simulink model "MPC_DUE"  (R2019a)
settings: Solver=FixedStepAuto  StartTime=0.0  StopTime=120  RelTol=1e-3  EnableMultiTasking=on
undefined symbols (not defined in the file or in its folder): DiscIntNeverNeededParam, i0, sigbuilder_block, Ts, u0, y0
libraries: MagnetoLibrary x3
settings Model: SimulationMode=external  ExtModeTrigDuration=2  Creator=jakub  LastModifiedBy=jakub
settings OptimizationCC: EnhancedBackFolding=on  PassReuseOutputArgsAs=Individual arguments  MaxStackSize=64  OptimizeBlockOrder=speed  DifferentSizesBufferReuse=on  OptimizationCustomize=off
settings DebuggingCC: ParameterTunabilityLossMsg=error
settings HardwareCC: ProdBitPerPointer=32  ProdBitPerSizeT=32  ProdBitPerPtrDiffT=32  ProdLargestAtomicInteger=Long  ProdLargestAtomicFloat=Double  ProdWordSize=32  ProdHWDeviceType=ARM Compatible->ARM Cortex
settings SFSimCC: MATLABDynamicMemAlloc=off
settings RTWCC: SystemTargetFile=ert.tlc  HardwareBoard=Arduino Due  TLCOptions=-aInlineSetEventsForThisBaseRateFcn=TLC_FALSE -aSuppressMultiTaskScheduler=TLC_FALSE -aRateBasedStepFcn=1  TemplateMakefile=ert_default_tmf  GenerateReport=on  Toolchain=Arduino ARM  BuildConfiguration=Faster Runs  IncludeHyperlinkInReport=on  LaunchReport=on  GenerateTraceInfo=on  GenerateTraceReport=on  GenerateTraceReportSl=on  GenerateTraceReportSf=on  GenerateTraceReportEml=on
settings CodeAppCC: ForceParamTrailComments=on  IgnoreCustomStorageClasses=off  OperatorAnnotations=on  SimulinkDataObjDesc=on  SFDataObjDesc=on  InsertBlockDesc=on
settings ERTTargetCC: SupportContinuousTime=on  SupportVariableSizeSignals=on  ExtModeStaticAllocSize=24576

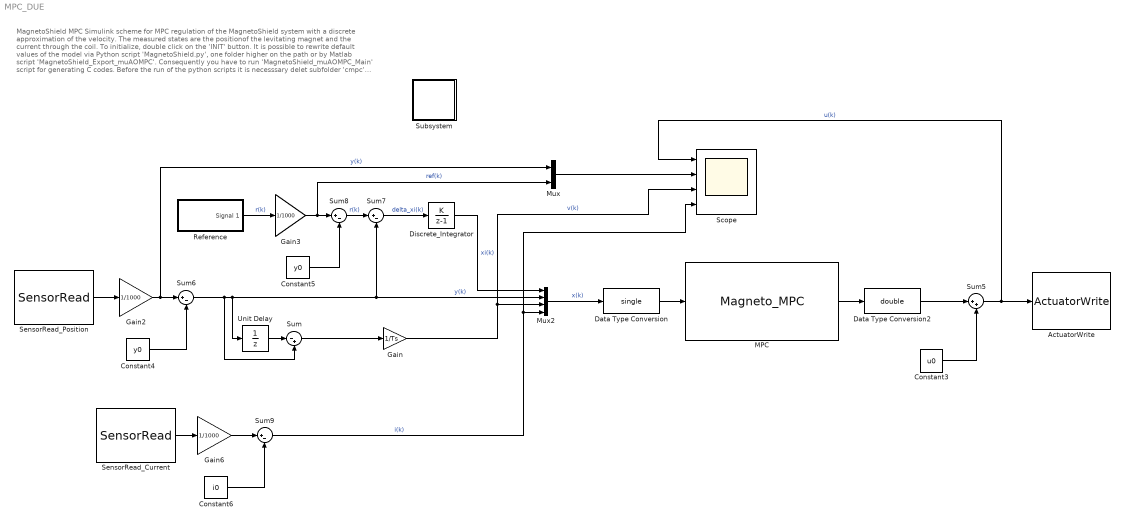
== system MPC_DUE ==
  note: MagnetoShield MPC
      | Simulink scheme for MPC regulation of the MagnetoShield system with a discrete approximation of the velocity.
      | The measured states are the positionof the levitating magnet and the current through the coil.
      | To initialize, double click on the 'INIT' button.
      |
      | It is possible to rewrite default values of the model via Python script 'MagnetoShield.py', one folder higher on
      | the path or by Matlab script 'MagnetoShield_Export_muAOMPC'.
      | Consequently you have to run 'MagnetoShield_muAOMPC_Main' script for generating C codes. Before the run
      | of the python scripts it is necesssary delet subfolder 'cmpc' (will be regenerated). If the application performance
      | did not change, errase all files in the subfolder '.../MagnetoShield_MPC_DUE/MagnetoShield_MPC_Control' too
      | and in 'MPC' block build the S-Function again.
      |
      | For a correct performance of the control-loop it is necessary to have '.../MagnetoShield_MPC_DUE/cmpc' folder
      | added in the Matlab path.
  ActuatorWrite : MagnetoLibrary/ActuatorWrite  Board=DUE  Units=Volts
      settings: SourceProductName=AutomationShield
  Constant3 : Constant  Value=u0
  Constant4 : Constant  Value=y0
  Constant5 : Constant  Value=y0
  Constant6 : Constant  Value=i0
  Data Type Conversion : DataTypeConversion  OutDataTypeStr=single
  Data Type Conversion2 : DataTypeConversion  OutDataTypeStr=double
  Discrete_Integrator : DiscreteIntegrator  IntegratorMethod=Accumulation: Forward Euler  SampleTime=Ts  LimitOutput=on  UpperSaturationLimit=100  LowerSaturationLimit=-100  ICPrevOutput=DiscIntNeverNeededParam  ICPrevScaledInput=DiscIntNeverNeededParam
  Gain : Gain  Gain=1/Ts
  Gain2 : Gain  Gain=1/1000
  Gain3 : Gain  Gain=1/1000
  Gain6 : Gain  Gain=1/1000
  MPC : S-Function  InitFcn=try, set_param(gcb,'FunctionName','Magneto_MPC'), end  FunctionName=Magneto_MPC  SFunctionModules=Magneto_MPC_wrapper mtx_ops mpc_const mpc mpc_ref mpc_stc mpc_inc fip_ops  SFunctionDeploymentMode=off  EnableBusSupport=off  mask(S-Function Builder){}
      mask help: Simulink:masks:SFunctionBuilder_MD
      mask init:
      | val = [[.9  0.75 0.75 1 1 .9 .9 1]',[1 1 0.75 0.75 .9 .9 1 .9]'];try , sys = get_param(gcb,'SfunBuilderFcnName');if isempty(sys), sys = get_param(gcb,'FunctionName'); end,catch, sys = get_param(gcb,'FunctionName'); end
      settings: CopyFcn=set_param(gcbh,'LinkStatus','none')  PreSaveFcn=try, set_param(gcb,'FunctionName','Magneto_MPC'), end  OpenFcn=sfunctionwizard(gcbh)
      mask Display: plot(val(:,1),val(:,2)),disp(sys), port_label('input',1,'u'), port_label('output',1,'y')
  Mux : Mux  Inputs=2
  Mux2 : Mux
  Reference : Subsystem  Tag=STV Subsys  LoadFcn=sigbuilder_block('load');  StartFcn=sigbuilder_block('start');  StopFcn=sigbuilder_block('stop');  ClipboardFcn=sigbuilder_block('clipboard');  mask(Sigbuilder block){tuvar=[0:10]}
      mask help: Simulink:masks:SigbuilderBlock_MD
      mask init:
      | if ~strcmp(get_param(bdroot(gcbh),'SimulationStatus'),'stopped') tuvar = sigbuilder_block('maskInit'); end
      settings: CopyFcn=sigbuilder_block('copy');  DeleteFcn=sigbuilder_block('delete');  ModelCloseFcn=sigbuilder_block('modelClose');  PreSaveFcn=sigbuilder_block('preSave');  PauseFcn=sigbuilder_block('pause');  ContinueFcn=sigbuilder_block('continue');  NameChangeFcn=sigbuilder_block('namechange');  OpenFcn=sigbuilder_block('open',[61.8 52.2 1012.8 447.6 ]);  CloseFcn=sigbuilder_block('close');
      mask Display: plot(0, 0, 100, 100,[2, 2, 32, 32, 2], [68, 8, 8, 68, 68],[32, 2], [38, 38], [32, 19, 2],[53, 60, 44], [32, 17, 17, 2],[16, 16, 31, 31]);txt = getActiveGroup(gcbh);text(2, 100, txt,'verticalAlignment', 'top');
  Scope : Scope  NumInputPorts=4
  SensorRead_Current : MagnetoLibrary/SensorRead  board=DUE  sensor=Current [mA]  sampling=Ts
      settings: SourceProductName=AutomationShield
  SensorRead_Position : MagnetoLibrary/SensorRead  board=DUE  sensor=Distance [mm]  sampling=Ts
      settings: SourceProductName=AutomationShield
  Subsystem : Subsystem
      settings: OpenFcn=|
      | clear;close all;clc;
      | cd(fileparts(which(gcs)));
      | load '../../../../../../matlab/examples/MagnetoShield/MagnetoShield_Models_Greybox_SS';
      | 
      | Ts = 0.003
      mask Display: disp('INIT')
  Sum : Sum  Inputs=|-+
  Sum5 : Sum  Inputs=|++
  Sum{6..9} (4 alike) : Sum  Inputs=|+-
  Unit Delay : UnitDelay  SampleTime=-1  HasFrameUpgradeWarning=on
  wires:
  SensorRead_Current/1 -> Gain6/1
  Discrete_Integrator/1 -> Mux2/1  "xi(k)"
  Unit Delay/1 -> Sum/1
  Sum/1 -> Gain/1
  Gain3/1 -> Mux/2, Sum8/1  "ref(k)"
  Constant5/1 -> Sum8/2
  Constant6/1 -> Sum9/2
  Gain/1 -> Mux2/3, Scope/3  "v(k)"
  Reference/1(Signal 1) -> Gain3/1  "r(k)"
  Sum8/1 -> Sum7/1  "r(k)"
  Constant4/1 -> Sum6/2
  Sum7/1 -> Discrete_Integrator/1  "delta_xi(k)"
  Gain2/1 -> Mux/1, Sum6/1  "y(k)"
  Gain6/1 -> Sum9/1
  SensorRead_Position/1 -> Gain2/1
  Sum9/1 -> Mux2/4, Scope/4  "i(k)"
  Sum6/1 -> Sum/2, Unit Delay/1, Mux2/2, Sum7/2  "y(k)"
  Sum5/1 -> ActuatorWrite/1, Scope/1  "u(k)"
  Constant3/1 -> Sum5/2
  Mux2/1 -> Data Type Conversion/1  "x(k)"
  Data Type Conversion/1 -> MPC/1
  MPC/1 -> Data Type Conversion2/1
  Data Type Conversion2/1 -> Sum5/1
  Mux/1 -> Scope/2

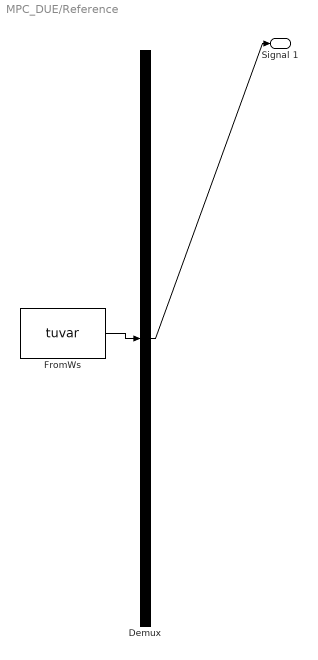
== system MPC_DUE/Reference ==
  Demux : Demux  Tag=STV Demux  Outputs=1
  FromWs : FromWorkspace  Tag=STV FromWs  VariableName=tuvar  SampleTime=0
      SigBuilderData=|
      | common.afterFinalStr = 'Extrapolate'
      | common.sampleTime = 0
      | dataSet.timeRange = [0 120]
      | dataSet.name = 'Group 1'
      | sbobj.Groups.Name = 'Group 1'
      | sbobj.Groups.Signals.Name = 'Signal 1'
      | sbobj.Groups.Signals.XData = [0 5 5 10 15 15 20 25 25 30 35 35 40 45 45 50 55 55 60 65 70 70 75 80 85 85 90 95 100 105 110 115 115 120]
      | sbobj.Groups.Signals.YData = [17 17 16.5 16.5 16.5 15.5 15.5 15.5 14.5 14.5 14.5 13.5 13.5 13.5 12.5 12.5 12.5 16 16 16 16 13.5 13.5 13.5 13.5 15 15 15 17 12 14.5 14.5 17 17]
      | sbobj.Groups.TimeRange = [0 120]
  Signal 1 : Outport  Tag=STV Outport
  wires:
  FromWs/1 -> Demux/1
  Demux/1 -> Signal 1/1

== system MPC_DUE/Subsystem ==
